simulink model "Simulaciones_lab_1sirve"  (R2024b)
settings: Solver=VariableStepAuto  StartTime=0.0  StopTime=50  RelTol=1e-3
values from neighbouring files (symbols this model uses):
  A_cc = T_cc_inv*matA*T_cc    [simulation.m]
  A_co = T_co_inv*matA*T_co    [simulation.m]
  B_cc = T_cc_inv*matB    [simulation.m]
  B_co = T_co_inv*matB    [simulation.m]
  C_cc = matC*T_cc    [simulation.m]
  C_co = matC*T_co    [simulation.m]
  D_cc = matD    (= 0)    [simulation.m]
  D_co = matD    (= 0)    [simulation.m]
  E_cc = T_cc_inv * matE    [simulation.m]
  E_co = T_co_inv * matE    [simulation.m]
  F_cc = matF    (= 0)    [simulation.m]
  F_co = matF    (= 0)    [simulation.m]
  K_cc_m1 = double(subs(K_vec_sym, res_cc))    [simulation.m]
  K_cc_m3 = K_ack_cc(1:end-1)    [simulation.m]
  K_co_m1 = double(subs(K_vec_sym, res_co))    [simulation.m]
  K_co_m3 = K_ack_co(1:end-1)    [simulation.m]
  K_std_m3 = K_ack_std(1:end-1)    [simulation.m]
  Ki_cc_m1 = double(res_cc.Ki_sym)    [simulation.m]
  Ki_cc_m3 = -K_ack_cc(end)    [simulation.m]
  Ki_co_m1 = double(res_co.Ki_sym)    [simulation.m]
  Ki_co_m3 = -K_ack_co(end)    [simulation.m]
  Ki_std_m3 = -K_ack_std(end)    [simulation.m]
  matA = zeros(3,3)    [post_process.m]    (also in simulation.m)
  matB = zeros(3,1); matB(2,1) = -(2*Ir*Km)/a; matB(3,1) = Km    [post_process.m]    (also in simulation.m = zeros(3,1))
  matC = [1,0,0]    [post_process.m]    (also in simulation.m = [1, 0, 0])
  matD = 0    [post_process.m]    (also in simulation.m)
  matE = zeros(3,1)    [simulation.m]
  matF = 0    [simulation.m]
undefined symbols (not defined in the file or in its folder): K_cc_m2, K_co_m2, K_std_m2, Ki_cc_m2, Ki_co_m2, Ki_std_m2

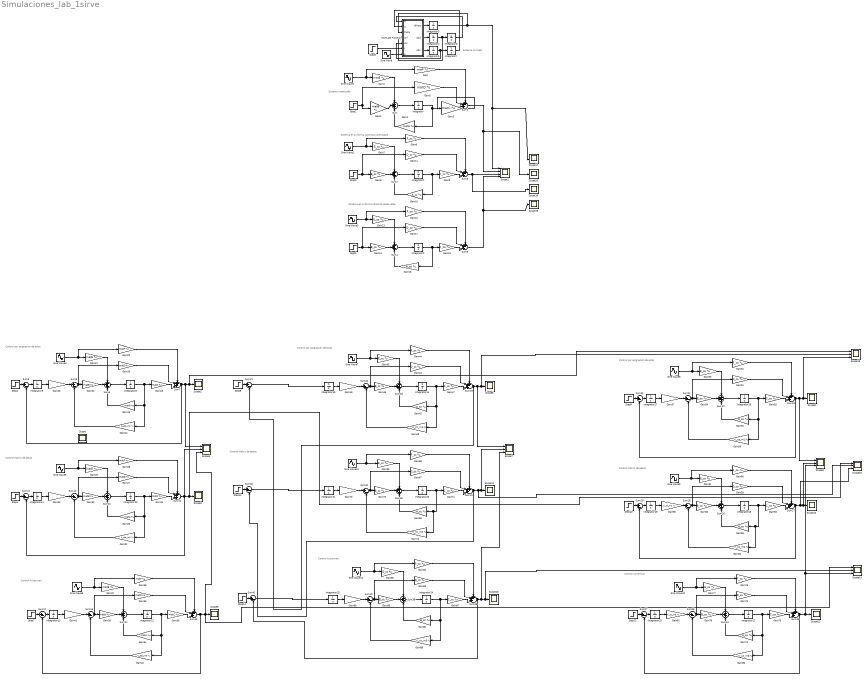
== system Simulaciones_lab_1sirve ==
  note: Sistema no lineal
  note: Sistema en su forma canonica observable
  note: Sistema en su forma canonica controlable
  note: Sistema linealizado
  note: Control por asignación de polos
  note: Control Matriz de pesos
  note: Control Ackerman
  note: Control por asignación de polos
  note: Control por asignación de polos
  note: Control Matriz de pesos
  note: Control Matriz de pesos
  note: Control Ackerman
  note: Control Ackerman
  Gain{,20,28,36} (4 alike) : Gain  Gain=matF  Multiplication=Matrix(K*u)
  Gain{1,21,29,37} (4 alike) : Gain  Gain=matE  Multiplication=Matrix(K*u)
  Gain{10,42,66,82} (4 alike) : Gain  Gain=A_cc  Multiplication=Matrix(K*u)
  Gain{11,43,67,83} (4 alike) : Gain  Gain=D_cc  Multiplication=Matrix(K*u)
  Gain{12,52,60,76} (4 alike) : Gain  Gain=F_co  Multiplication=Matrix(K*u)
  Gain{13,53,61,77} (4 alike) : Gain  Gain=E_co  Multiplication=Matrix(K*u)
  Gain{14,54,62,78} (4 alike) : Gain  Gain=B_co  Multiplication=Matrix(K*u)
  Gain{15,55,63,79} (4 alike) : Gain  Gain=C_co  Multiplication=Matrix(K*u)
  Gain{16,50,58,74} (4 alike) : Gain  Gain=A_co  Multiplication=Matrix(K*u)
  Gain{17,51,59,75} (4 alike) : Gain  Gain=D_co  Multiplication=Matrix(K*u)
  Gain{4,18,26,34} (4 alike) : Gain  Gain=matA  Multiplication=Matrix(K*u)
  Gain{5,19,27,35} (4 alike) : Gain  Gain=matD  Multiplication=Matrix(K*u)
  Gain{2,22,30,38} (4 alike) : Gain  Gain=matB  Multiplication=Matrix(K*u)
  Gain{3,23,31,39} (4 alike) : Gain  Gain=matC  Multiplication=Matrix(K*u)
  Gain24 : Gain  Gain=K_std_m2  Multiplication=Matrix(K*u)
  Gain25 : Gain  Gain=Ki_std_m2  Multiplication=Matrix(K*u)
  Gain32 : Gain  Gain=K_std_m2  Multiplication=Matrix(K*u)
  Gain33 : Gain  Gain=Ki_std_m2  Multiplication=Matrix(K*u)
  Gain40 : Gain  Gain=K_std_m3  Multiplication=Matrix(K*u)
  Gain41 : Gain  Gain=Ki_std_m3  Multiplication=Matrix(K*u)
  Gain{6,44,68,84} (4 alike) : Gain  Gain=F_cc  Multiplication=Matrix(K*u)
  Gain{7,45,69,85} (4 alike) : Gain  Gain=E_cc  Multiplication=Matrix(K*u)
  Gain{8,46,70,86} (4 alike) : Gain  Gain=B_cc  Multiplication=Matrix(K*u)
  Gain{9,47,71,87} (4 alike) : Gain  Gain=C_cc  Multiplication=Matrix(K*u)
  Gain48 : Gain  Gain=K_cc_m1  Multiplication=Matrix(K*u)
  Gain49 : Gain  Gain=Ki_cc_m1  Multiplication=Matrix(K*u)
  Gain56 : Gain  Gain=K_co_m1  Multiplication=Matrix(K*u)
  Gain57 : Gain  Gain=Ki_co_m1  Multiplication=Matrix(K*u)
  Gain64 : Gain  Gain=K_co_m2  Multiplication=Matrix(K*u)
  Gain65 : Gain  Gain=Ki_co_m2  Multiplication=Matrix(K*u)
  Gain72 : Gain  Gain=K_cc_m2  Multiplication=Matrix(K*u)
  Gain73 : Gain  Gain=Ki_cc_m2  Multiplication=Matrix(K*u)
  Gain80 : Gain  Gain=K_co_m3  Multiplication=Matrix(K*u)
  Gain81 : Gain  Gain=Ki_co_m3  Multiplication=Matrix(K*u)
  Gain88 : Gain  Gain=K_cc_m3  Multiplication=Matrix(K*u)
  Gain89 : Gain  Gain=Ki_cc_m3  Multiplication=Matrix(K*u)
  Integrator{,1..25} (26 alike) : Integrator
  MATLAB Function : MATLAB Function  TreatAsAtomicUnit=on
  Scope1 : Scope  NumInputPorts=4
  Scope{,2..3,5..6,8,10..13,17..20} (14 alike) : Scope
  Scope{4,7,9,14..16} (6 alike) : Scope  NumInputPorts=3
  Sine Wave{,1..3} (4 alike) : Sin  Amplitude=0.1  SampleTime=0
  Sine Wave{4..12} (9 alike) : Sin  Amplitude=0.000001  SampleTime=0
  Step{1,3,5..6} (4 alike) : Step  After=25  SampleTime=0
  Step{2,4,7..13} (9 alike) : Step  Time=5  After=5  SampleTime=0
  Sum{,2,4,6,10,14,18,22,26,30,34,38} (12 alike) : Sum  Inputs=+++
  Sum{1,3,5,7,11,15,19,23,27,31,35,39} (12 alike) : Sum  Inputs=+++|
  Sum{8..9,12..13,16..17,20..21,24..25,28..29,32..33,36..37,40..41} (18 alike) : Sum  Inputs=|+-
  wires:
  Gain2/1 -> Sum/2
  Gain4/1 -> Sum/3
  Sum/1 -> Integrator/1
  Integrator/1 -> Gain4/1, Gain3/1
  Gain/1 -> Sum1/1
  Gain5/1 -> Sum1/2
  Gain3/1 -> Sum1/3
  Step1/1 -> Gain5/1, Gain2/1
  Sine Wave1/1 -> Gain/1, Gain1/1
  Gain1/1 -> Sum/1
  Sum1/1 -> Scope1/2, Scope20/1
  Gain7/1 -> Sum2/1
  Gain10/1 -> Sum2/3
  Sine Wave2/1 -> Gain6/1, Gain7/1
  Gain9/1 -> Sum3/3
  Gain6/1 -> Sum3/1
  Gain11/1 -> Sum3/2
  Step3/1 -> Gain11/1, Gain8/1
  Sum2/1 -> Integrator1/1
  Gain8/1 -> Sum2/2
  Integrator1/1 -> Gain10/1, Gain9/1
  Gain13/1 -> Sum4/1
  Gain16/1 -> Sum4/3
  Sine Wave3/1 -> Gain12/1, Gain13/1
  Gain15/1 -> Sum5/3
  Gain12/1 -> Sum5/1
  Gain17/1 -> Sum5/2
  Step5/1 -> Gain17/1, Gain14/1
  Sum4/1 -> Integrator2/1
  Gain14/1 -> Sum4/2
  Integrator2/1 -> Gain16/1, Gain15/1
  Sum3/1 -> Scope18/1, Scope1/3
  Sum5/1 -> Scope1/4, Scope19/1
  Step6/1 -> MATLAB Function/6(f)
  MATLAB Function/1(dtheta) -> Integrator3/1
  MATLAB Function/2(ddxf) -> Integrator4/1
  MATLAB Function/3(ddxr) -> Integrator5/1
  Integrator4/1 -> MATLAB Function/4(dxf), Integrator6/1
  Integrator5/1 -> MATLAB Function/5(dxr), Integrator7/1
  Integrator3/1 -> Scope1/1, Scope17/1, MATLAB Function/3(theta)
  Integrator6/1 -> MATLAB Function/1(xf)
  Integrator7/1 -> MATLAB Function/2(xr)
  Sine Wave/1 -> MATLAB Function/7(p)
  Gain19/1 -> Sum7/2
  Sum6/1 -> Integrator8/1
  Gain22/1 -> Sum6/2
  Gain23/1 -> Sum7/3
  Gain21/1 -> Sum6/1
  Sum7/1 -> Scope4/1, Scope15/1, Scope2/1, Sum9/2
  Gain18/1 -> Sum6/3
  Sine Wave4/1 -> Gain20/1, Gain21/1
  Gain20/1 -> Sum7/1
  Integrator8/1 -> Gain24/1, Gain18/1, Gain23/1
  Sum8/1 -> Gain19/1, Gain22/1
  Integrator9/1 -> Gain25/1
  Gain25/1 -> Sum8/1
  Gain24/1 -> Sum8/2
  Step2/1 -> Sum9/1
  Sum9/1 -> Integrator9/1
  Sum13/1 -> Integrator11/1
  Step4/1 -> Sum13/1
  Gain32/1 -> Sum12/2
  Integrator11/1 -> Gain33/1
  Gain33/1 -> Sum12/1
  Gain28/1 -> Sum11/1
  Sine Wave5/1 -> Gain28/1, Gain29/1
  Gain26/1 -> Sum10/3
  Sum11/1 -> Scope4/2, Scope16/1, Scope3/1, Sum13/2
  Gain29/1 -> Sum10/1
  Integrator10/1 -> Gain32/1, Gain26/1, Gain31/1
  Sum12/1 -> Gain27/1, Gain30/1
  Gain27/1 -> Sum11/2
  Gain30/1 -> Sum10/2
  Sum10/1 -> Integrator10/1
  Gain31/1 -> Sum11/3
  Sum14/1 -> Integrator12/1
  Sine Wave6/1 -> Gain36/1, Gain37/1
  Integrator12/1 -> Gain40/1, Gain34/1, Gain39/1
  Gain34/1 -> Sum14/3
  Gain37/1 -> Sum14/1
  Gain39/1 -> Sum15/3
  Sum15/1 -> Scope4/3, Scope14/1, Scope5/1, Sum17/2
  Gain38/1 -> Sum14/2
  Gain36/1 -> Sum15/1
  Integrator13/1 -> Gain41/1
  Sum17/1 -> Integrator13/1
  Gain41/1 -> Sum16/1
  Gain40/1 -> Sum16/2
  Step7/1 -> Sum17/1
  Sum16/1 -> Gain35/1, Gain38/1
  Gain35/1 -> Sum15/2
  Sum19/1 -> Scope7/1, Scope15/2, Scope6/1, Sum21/2
  Sum18/1 -> Integrator14/1
  Gain44/1 -> Sum19/1
  Gain49/1 -> Sum20/1
  Gain46/1 -> Sum18/2
  Sine Wave7/1 -> Gain44/1, Gain45/1
  Sum20/1 -> Gain43/1, Gain46/1
  Integrator15/1 -> Gain49/1
  Gain48/1 -> Sum20/2
  Sum21/1 -> Integrator15/1
  Gain42/1 -> Sum18/3
  Gain47/1 -> Sum19/3
  Integrator14/1 -> Gain48/1, Gain42/1, Gain47/1
  Step8/1 -> Sum21/1
  Gain45/1 -> Sum18/1
  Gain43/1 -> Sum19/2
  Gain53/1 -> Sum22/1
  Integrator16/1 -> Gain56/1, Gain50/1, Gain55/1
  Gain50/1 -> Sum22/3
  Gain55/1 -> Sum23/3
  Gain57/1 -> Sum24/1
  Sum25/1 -> Integrator17/1
  Integrator17/1 -> Gain57/1
  Sum23/1 -> Scope9/1, Scope15/3, Scope8/1, Sum25/2
  Step9/1 -> Sum25/1
  Sum22/1 -> Integrator16/1
  Gain52/1 -> Sum23/1
  Gain54/1 -> Sum22/2
  Sine Wave8/1 -> Gain52/1, Gain53/1
  Sum24/1 -> Gain51/1, Gain54/1
  Gain56/1 -> Sum24/2
  Gain51/1 -> Sum23/2
  Gain62/1 -> Sum26/2
  Sine Wave9/1 -> Gain61/1, Gain60/1
  Gain60/1 -> Sum27/1
  Sum27/1 -> Scope16/3, Scope9/2, Scope10/1, Sum29/2
  Gain59/1 -> Sum27/2
  Gain64/1 -> Sum28/2
  Step10/1 -> Sum29/1
  Gain61/1 -> Sum26/1
  Gain65/1 -> Sum28/1
  Sum26/1 -> Integrator18/1
  Gain58/1 -> Sum26/3
  Integrator18/1 -> Gain64/1, Gain58/1, Gain63/1
  Sum28/1 -> Gain59/1, Gain62/1
  Sum29/1 -> Integrator19/1
  Gain63/1 -> Sum27/3
  Integrator19/1 -> Gain65/1
  Gain68/1 -> Sum31/1
  Gain71/1 -> Sum31/3
  Sum31/1 -> Scope16/2, Scope7/2, Scope11/1, Sum33/2
  Sum33/1 -> Integrator21/1
  Gain66/1 -> Sum30/3
  Gain67/1 -> Sum31/2
  Sum30/1 -> Integrator20/1
  Gain72/1 -> Sum32/2
  Integrator20/1 -> Gain72/1, Gain66/1, Gain71/1
  Step11/1 -> Sum33/1
  Gain70/1 -> Sum30/2
  Gain73/1 -> Sum32/1
  Sum32/1 -> Gain67/1, Gain70/1
  Sine Wave10/1 -> Gain69/1, Gain68/1
  Gain69/1 -> Sum30/1
  Integrator21/1 -> Gain73/1
  Integrator25/1 -> Gain89/1
  Step13/1 -> Sum41/1
  Integrator24/1 -> Gain88/1, Gain82/1, Gain87/1
  Gain86/1 -> Sum38/2
  Gain85/1 -> Sum38/1
  Sine Wave11/1 -> Gain84/1, Gain85/1
  Sum39/1 -> Scope7/3, Scope14/2, Scope13/1, Sum41/2
  Sum38/1 -> Integrator24/1
  Gain83/1 -> Sum39/2
  Gain82/1 -> Sum38/3
  Gain84/1 -> Sum39/1
  Gain79/1 -> Sum35/3
  Gain74/1 -> Sum34/3
  Gain89/1 -> Sum40/1
  Integrator23/1 -> Gain81/1
  Integrator22/1 -> Gain80/1, Gain74/1, Gain79/1
  Gain87/1 -> Sum39/3
  Sum37/1 -> Integrator23/1
  Sum40/1 -> Gain83/1, Gain86/1
  Gain81/1 -> Sum36/1
  Sum35/1 -> Scope14/3, Scope9/3, Scope12/1, Sum37/2
  Sine Wave12/1 -> Gain76/1, Gain77/1
  Step12/1 -> Sum37/1
  Gain80/1 -> Sum36/2
  Sum34/1 -> Integrator22/1
  Sum36/1 -> Gain75/1, Gain78/1
  Gain76/1 -> Sum35/1
  Gain77/1 -> Sum34/1
  Gain88/1 -> Sum40/2
  Gain75/1 -> Sum35/2
  Sum41/1 -> Integrator25/1
  Gain78/1 -> Sum34/2

== matlab function Simulaciones_lab_1sirve/MATLAB Function ==
function [dtheta, ddxf, ddxr]=fcn(xf, xr, theta, dxf, dxr, f, p)

g = 9.81;        % m/s^2
mf = 30;         % kg
mr = 50;         % kg
kf  = 10000;     % N/m
kr  = 15000;     % N/m
ksf = 19500;     % N/m
ksr = 12500;     % N/m
bsf = 1000;      % Ns/m
bsr = 1100;      % Ns/m
a = 0.8;         % m
b = 0.7;         % m
c = 0.5;         % m

dtheta = (- f*c - ksf*xf*a - ksf*a^2*theta + ksr*xr*b - ksr*b^2*theta + bsr*dxr*b + bsf*dxf*a)/(bsr*b^2 + bsf*a^2)
ddxf = (- mf*g - kf*xf + kf*p - ksf*xf - ksf*a*theta - bsf*dxf - bsf*a*dtheta)/mf
ddxr = (- mr*g - kr*xr - ksr*xr + ksr*b*theta - bsr*dxr + bsr*b*dtheta)/mr

 ;
